simulink model "altitude_smoothening"  (R2025b)
settings: Solver=FixedStepDiscrete  StartTime=0.0  StopTime=10.0  FixedStep=0.1  RelTol=1e-3
settings OptimizationCC: DefaultParameterBehavior=Inlined  EnhancedBackFolding=on  PassReuseOutputArgsAs=Individual arguments  ZeroExternalMemoryAtStartup=off  ZeroInternalMemoryAtStartup=off  OptimizeBlockOrder=speed  DifferentSizesBufferReuse=on  OptimizationCustomize=off  EfficientTunableParamExpr=on
settings DebuggingCC: ParameterTunabilityLossMsg=error
settings SFSimCC: MATLABDynamicMemAlloc=off
settings RTWCC: SystemTargetFile=ert.tlc  GenCodeOnly=on  TemplateMakefile=ert_default_tmf  Description=Embedded Coder
settings CodeAppCC: ForceParamTrailComments=on  IgnoreCustomStorageClasses=off  MaxIdLength=128.0  OperatorAnnotations=on  SimulinkDataObjDesc=on  SFDataObjDesc=on  InsertBlockDesc=on  InternalIdentifier=Classic
settings ERTTargetCC: ERTCustomFileTemplate=example_file_process.tlc  TargetLangStandard=C99 (ISO)  GenerateSampleERTMain=on

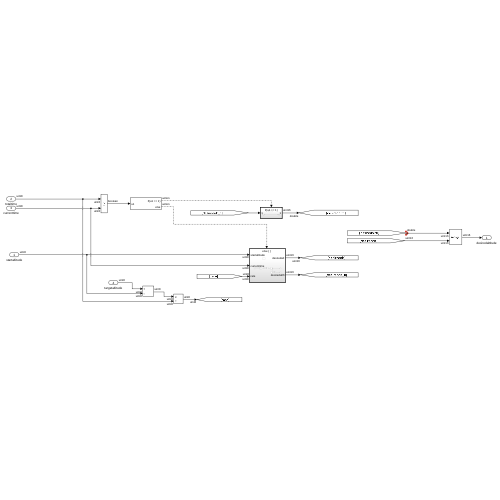
[thumbnail: Simulink's stored preview of the top-level diagram]
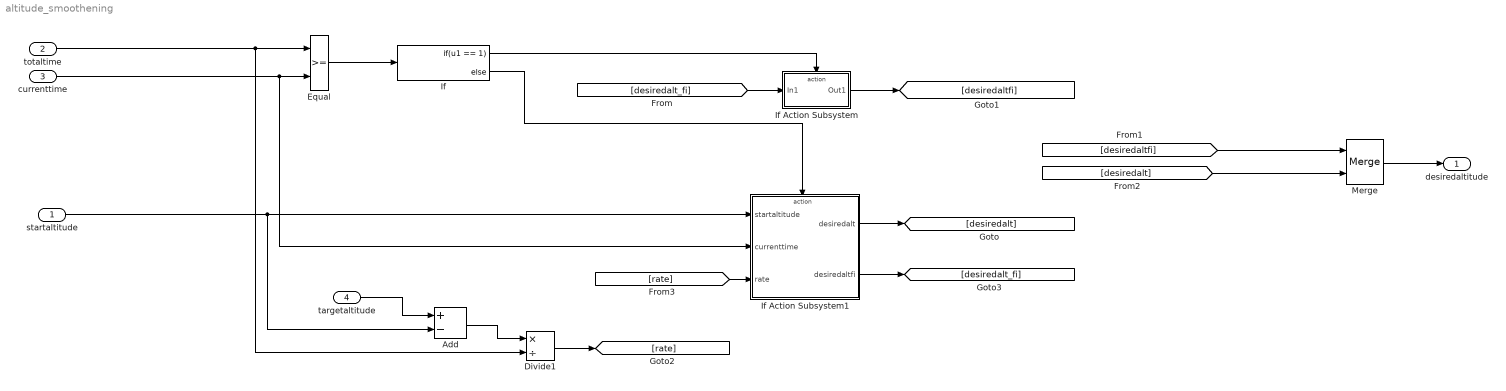
== system altitude_smoothening ==
  startaltitude : Inport  OutDataTypeStr=uint8
  totaltime : Inport  Port=2  OutDataTypeStr=uint8
  currenttime : Inport  Port=3  OutDataTypeStr=uint8
  targetaltitude : Inport  Port=4  OutDataTypeStr=uint8
  Add : Sum  Inputs=+-
  Divide1 : Product  Inputs=*/
  Equal : RelationalOperator  OutDataTypeStr=boolean  RndMeth=Simplest  InputSameDT=off
  If : If  IfExpression=u1 == 1
  If Action Subsystem : Subsystem  TreatAsAtomicUnit=on
  If Action Subsystem1 : Subsystem  TreatAsAtomicUnit=on
  Merge : Merge
  desiredaltitude : Outport
  wires:
  currenttime/1 -> If Action Subsystem1/2(currenttime), Equal/2
  Equal/1 -> If/1
  If/1 -> If Action Subsystem/Action
  If Action Subsystem/1(Out1) -> [desiredaltfi]
  If/2 -> If Action Subsystem1/Action
  Merge/1 -> desiredaltitude/1
  [desiredalt_fi] -> If Action Subsystem/1(In1)
  targetaltitude/1 -> Add/1
  startaltitude/1 -> If Action Subsystem1/1(startaltitude), Add/2
  Add/1 -> Divide1/1
  totaltime/1 -> Divide1/2, Equal/1
  Divide1/1 -> [rate]
  [rate] -> If Action Subsystem1/3(rate)
  [desiredaltfi] -> Merge/1
  [desiredalt] -> Merge/2
  If Action Subsystem1/1(desiredalt) -> [desiredalt]
  If Action Subsystem1/2(desiredaltfi) -> [desiredalt_fi]

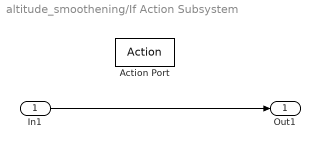
== system altitude_smoothening/If Action Subsystem ==
  In1 : Inport
  Action Port : ActionPort  ActionPortLabel=if(u1 == 1)
  Out1 : Outport  OutDataTypeStr=uint16
  wires:
  In1/1 -> Out1/1

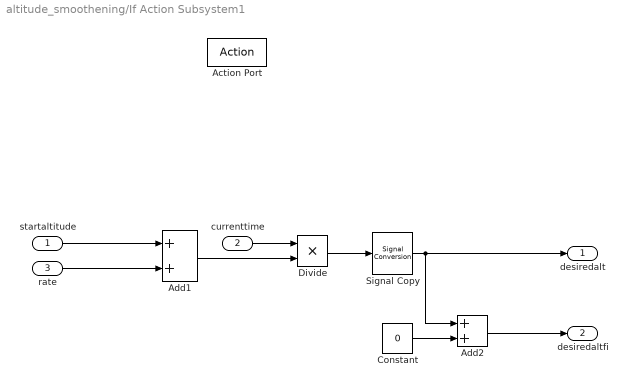
== system altitude_smoothening/If Action Subsystem1 ==
  startaltitude : Inport
  currenttime : Inport  Port=2
  rate : Inport  Port=3
  Action Port : ActionPort  ActionPortLabel=else
  Add1 : Sum
  Add2 : Sum
  Constant : Constant  Value=0  OutDataTypeStr=uint8
  Divide : Product  Inputs=**
  Signal Copy : SignalConversion  OverrideOpt=off
  desiredalt : Outport  OutDataTypeStr=uint16
  desiredaltfi : Outport  Port=2
  wires:
  startaltitude/1 -> Add1/1
  Add1/1 -> Divide/2
  currenttime/1 -> Divide/1
  rate/1 -> Add1/2
  Divide/1 -> Signal Copy/1
  Add2/1 -> desiredaltfi/1
  Constant/1 -> Add2/2
  Signal Copy/1 -> Add2/1, desiredalt/1
